simulink model "SetPointSimulink"  (R2020b)
settings: Solver=VariableStepAuto  StartTime=0.0  StopTime=10  RelTol=1e-3
values from neighbouring files (symbols this model uses):
  A = [-0.0558 -0.9968 0.0802 0.0415; 0.5980 -0.1150 -0.0318 0; -3.0500 0.3880 -0.4650 0; 0 0.0805 1 0]    [AircraftPaper.m]
  B = [0.0729 0; -4.7500 0.00775; 0.153 0.143; 0 0]    [AircraftPaper.m]
  C = [1 0 0 0; 0 0 0 1]    [AircraftPaper.m]
  F = inversa(1:4)    [AircraftPaper.m]
  Kc = lqr(A,B,Q,R)    [AircraftPaper.m]
  N = inversa(5:6)    [AircraftPaper.m]
  x0 = [pi/6 0 0 pi/4]    [AircraftPaper.m]
libraries: cstblocks x2
settings Model: Creator=leobartowski  LastModifiedBy=marydellarossa

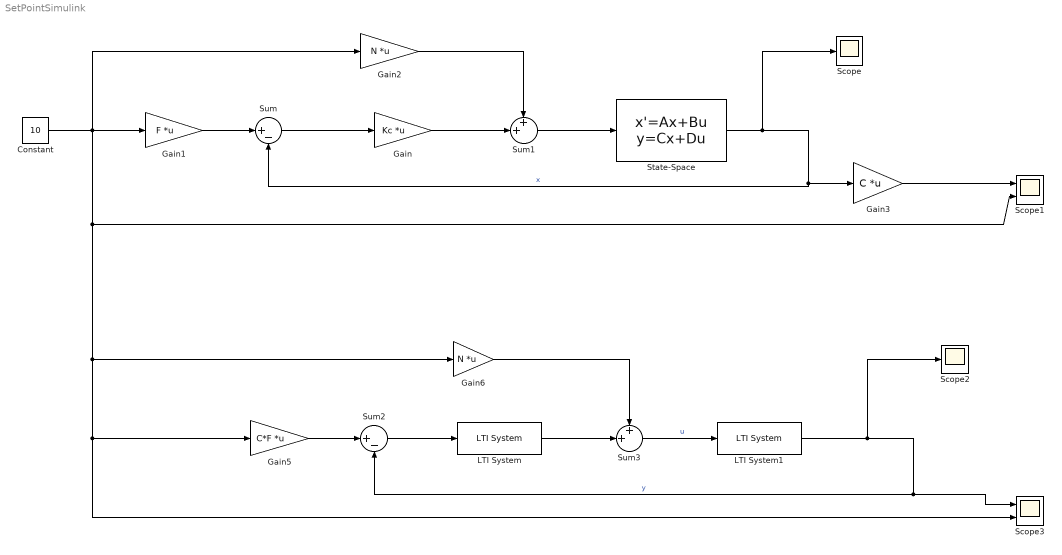
== system SetPointSimulink ==
  Constant : Constant  Value=10
  Gain : Gain  Gain=Kc  Multiplication=Matrix(K*u)
  Gain1 : Gain  Gain=F  Multiplication=Matrix(K*u)
  Gain2 : Gain  Gain=N  Multiplication=Matrix(K*u)
  Gain3 : Gain  Gain=C  Multiplication=Matrix(K*u)
  Gain5 : Gain  Gain=C*F  Multiplication=Matrix(K*u)
  Gain6 : Gain  Gain=N  Multiplication=Matrix(K*u)
  LTI System : cstblocks/LTI System  sys=K  IC=[]
  LTI System1 : cstblocks/LTI System  sys=Ps  IC=x0
  Scope : Scope
  Scope1 : Scope  NumInputPorts=2
  Scope2 : Scope
  Scope3 : Scope  NumInputPorts=2
  State-Space : StateSpace  A=A  B=B  C=eye(3)  D=zeros(3,1)  InitialCondition=x0
  Sum : Sum  Inputs=|+-
  Sum1 : Sum  Inputs=++|
  Sum2 : Sum  Inputs=|+-
  Sum3 : Sum  Inputs=++|
  wires:
  State-Space/1 -> Scope/1, Sum/2, Gain3/1  "x"
  Sum/1 -> Gain/1
  Gain/1 -> Sum1/2
  Sum1/1 -> State-Space/1
  Gain2/1 -> Sum1/1
  Gain1/1 -> Sum/1
  Gain3/1 -> Scope1/1
  LTI System/1 -> Sum3/2
  LTI System1/1 -> Scope2/1, Scope3/1, Sum2/2  "y"
  Sum2/1 -> LTI System/1
  Sum3/1 -> LTI System1/1  "u"
  Gain6/1 -> Sum3/1
  Constant/1 -> Gain2/1, Scope3/2, Gain5/1, Gain6/1, Scope1/2, Gain1/1
  Gain5/1 -> Sum2/1
